simulink model "Distribution_v1"  (Simulink 7.9)
settings: Solver=VariableStepDiscrete  StartTime=0.0  StopTime=500  RelTol=1e-3
libraries: simeventslib x13
(part 1 of 2)
settings Model: Creator=tsprock3  LastModifiedBy=tsprock3
settings DebuggingCC: SimStateOlderReleaseMsg=warning

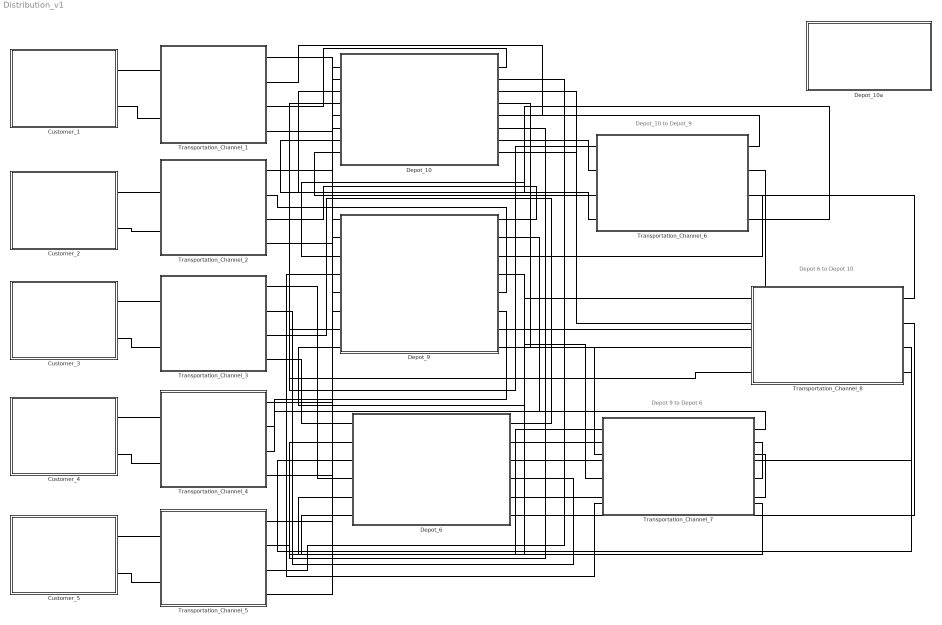
== system Distribution_v1 ==
  note: Depot_10 to Depot_9
  note: Depot 9 to Depot 6
  note: Depot 6 to Depot 10
  Customer_1 : Subsystem
  Customer_2 : Subsystem
  Customer_3 : Subsystem
  Customer_4 : Subsystem
  Customer_5 : Subsystem
  Depot_10 : Subsystem
  Depot_10a : Subsystem
  Depot_6 : Subsystem
  Depot_9 : Subsystem
  Transportation_Channel_1 : Subsystem
  Transportation_Channel_2 : Subsystem
  Transportation_Channel_3 : Subsystem
  Transportation_Channel_4 : Subsystem
  Transportation_Channel_5 : Subsystem
  Transportation_Channel_6 : Subsystem
  Transportation_Channel_7 : Subsystem
  Transportation_Channel_8 : Subsystem
  connections:
  Transportation_Channel_1/RConn4 -- Depot_10/LConn1
  Transportation_Channel_1/RConn3 -- Depot_10/RConn1
  Transportation_Channel_1/RConn1 -- Depot_10/LConn5
  Depot_10/RConn5 -- Transportation_Channel_1/RConn2
  Transportation_Channel_2/LConn2 -- Customer_2/RConn2
  Customer_2/RConn1 -- Transportation_Channel_2/LConn1
  Transportation_Channel_2/RConn1 -- Depot_9/LConn5
  Depot_9/RConn5 -- Transportation_Channel_2/RConn2
  Customer_3/RConn1 -- Transportation_Channel_3/LConn1
  Transportation_Channel_3/LConn2 -- Customer_3/RConn2
  Transportation_Channel_3/RConn1 -- Depot_6/LConn4
  Transportation_Channel_3/RConn2 -- Depot_6/RConn4
  Transportation_Channel_3/RConn3 -- Depot_6/RConn1
  Transportation_Channel_3/RConn4 -- Depot_6/LConn1
  Transportation_Channel_2/RConn3 -- Depot_9/RConn1
  Transportation_Channel_2/RConn4 -- Depot_9/LConn1
  Transportation_Channel_4/LConn2 -- Customer_4/RConn2
  Customer_4/RConn1 -- Transportation_Channel_4/LConn1
  Transportation_Channel_4/RConn1 -- Depot_9/LConn6
  Transportation_Channel_4/RConn3 -- Depot_9/RConn2
  Transportation_Channel_4/RConn4 -- Depot_9/LConn2
  Depot_9/RConn6 -- Transportation_Channel_4/RConn2
  Transportation_Channel_5/LConn2 -- Customer_5/RConn2
  Customer_5/RConn1 -- Transportation_Channel_5/LConn1
  Transportation_Channel_5/RConn1 -- Depot_10/LConn6
  Depot_10/RConn6 -- Transportation_Channel_5/RConn2
  Transportation_Channel_5/RConn3 -- Depot_10/RConn2
  Transportation_Channel_5/RConn4 -- Depot_10/LConn2
  Transportation_Channel_6/RConn3 -- Depot_9/RConn3
  Transportation_Channel_6/RConn4 -- Depot_9/LConn3
  Depot_10/RConn3 -- Transportation_Channel_6/LConn3
  Transportation_Channel_6/LConn4 -- Depot_10/LConn3
  Depot_6/RConn2 -- Transportation_Channel_7/RConn3
  Transportation_Channel_7/RConn4 -- Depot_6/LConn2
  Depot_9/RConn4 -- Transportation_Channel_7/LConn3
  Transportation_Channel_7/LConn4 -- Depot_9/LConn4
  Depot_6/RConn3 -- Transportation_Channel_8/RConn3
  Transportation_Channel_8/RConn4 -- Depot_6/LConn3
  Depot_10/LConn4 -- Transportation_Channel_8/LConn4
  Transportation_Channel_8/LConn3 -- Depot_10/RConn4
  Depot_10/RConn8 -- Transportation_Channel_8/LConn2
  Transportation_Channel_8/LConn1 -- Depot_6/LConn6
  Depot_6/RConn6 -- Transportation_Channel_8/RConn2
  Transportation_Channel_8/RConn1 -- Depot_10/LConn8
  Depot_10/RConn7 -- Transportation_Channel_6/LConn2
  Transportation_Channel_6/LConn1 -- Depot_9/LConn7
  Depot_9/RConn7 -- Transportation_Channel_6/RConn2
  Transportation_Channel_6/RConn1 -- Depot_10/LConn7
  Depot_9/RConn8 -- Transportation_Channel_7/LConn2
  Transportation_Channel_7/LConn1 -- Depot_6/LConn5
  Depot_6/RConn5 -- Transportation_Channel_7/RConn2
  Transportation_Channel_7/RConn1 -- Depot_9/LConn8
  Customer_1/RConn1 -- Transportation_Channel_1/LConn1
  Customer_1/RConn2 -- Transportation_Channel_1/LConn2

== system Distribution_v1/Customer_1 ==
  Clock : Clock
  Discrete Event Signal to Workspace : simeventslib/SimEvents Sinks/Discrete Event Signal to Workspace  VariableName=Customer_1  SaveFormat=Structure With Time  isMonitorOnly=off  isRecordIC=off
  Entity Sink : EntitySink
  Get Attribute : GetAttribute  AttributeName=Origin|Destination|Start  AttributeMissing=Error|Error|Error  AttributeDefaultValue=1|1|1  AttributeTreatAsVector=1|1|1  AttributeSendTiming=After entity departure|After entity departure|After entity departure  EvaluatedDefaultAttributeValue={[];[];[]}
      settings: OutputPortMap=o1,o2,o3
  Mux : Mux  Inputs=3
  Path Combiner : PathCombiner  NumberInputPorts=4
  Set Attribute : SetAttribute  AttributeName=Route|Origin|Destination|Start  AttributeFrom=Dialog|Dialog|Dialog|Signal port  AttributeValue=[1 10 9 2]|1|2|1  AttributeTreatAsVector=0|1|1|1  EvaluatedAttributeValue={[1 10 9 2];1;2;[]}
      settings: InputPortMap=u3
  Set Attribute1 : SetAttribute  AttributeName=Route|Origin|Destination|Start  AttributeFrom=Dialog|Dialog|Dialog|Signal port  AttributeValue=[1 10 6 3]|1|3|1  AttributeTreatAsVector=0|1|1|1  EvaluatedAttributeValue={[1 10 6 3];1;3;[]}
      settings: InputPortMap=u3
  Set Attribute2 : SetAttribute  AttributeName=Route|Origin|Destination|Start  AttributeFrom=Dialog|Dialog|Dialog|Signal port  AttributeValue=[1 10 5 0]|1|5|1  AttributeTreatAsVector=0|1|1|1  EvaluatedAttributeValue={[1 10 5 0];1;5;[]}
      settings: InputPortMap=u3
  Set Attribute3 : SetAttribute  AttributeName=Route|Origin|Destination|Start  AttributeFrom=Dialog|Dialog|Dialog|Signal port  AttributeValue=[1 10 9 4]|1|4|1  AttributeTreatAsVector=0|1|1|1  EvaluatedAttributeValue={[1 10 9 4];1;4;[]}
      settings: InputPortMap=u3
  Timed to Event Signal : TimedToEventSignal
  To_Customer_2 : TimeBasedEntityGenerator  Distribution=Exponential  InitialSeed=18340  Mean=1000/913  GenerateEntityAtSimulationStart=off
  To_Customer_3 : TimeBasedEntityGenerator  Distribution=Exponential  InitialSeed=13103  Mean=1000/105  GenerateEntityAtSimulationStart=off
  To_Customer_4 : TimeBasedEntityGenerator  Distribution=Exponential  InitialSeed=21557  Mean=1000/746  GenerateEntityAtSimulationStart=off
  To_Customer_5 : TimeBasedEntityGenerator  Distribution=Exponential  InitialSeed=24774  Mean=1000/737  GenerateEntityAtSimulationStart=off
  OUT_Shipment_1 : PMIOPort  Port=1  Side=Right
  IN_Shipment_1 : PMIOPort  Port=2  Side=Right
  wires:
  Clock/1 -> Timed to Event Signal/1
  Timed to Event Signal/1 -> Set Attribute/1, Set Attribute1/1, Set Attribute3/1, Set Attribute2/1
  Get Attribute/1 -> Mux/1
  Get Attribute/2 -> Mux/2
  Get Attribute/3 -> Mux/3
  Mux/1 -> Discrete Event Signal to Workspace/1
  connections:
  OUT_Shipment_1/RConn1 -- Path Combiner/RConn1
  To_Customer_2/RConn1 -- Set Attribute/LConn1
  To_Customer_3/RConn1 -- Set Attribute1/LConn1
  To_Customer_5/RConn1 -- Set Attribute2/LConn1
  To_Customer_4/RConn1 -- Set Attribute3/LConn1
  Set Attribute/RConn1 -- Path Combiner/LConn1
  Set Attribute1/RConn1 -- Path Combiner/LConn2
  Set Attribute3/RConn1 -- Path Combiner/LConn3
  Set Attribute2/RConn1 -- Path Combiner/LConn4
  Get Attribute/LConn1 -- IN_Shipment_1/RConn1
  Entity Sink/LConn1 -- Get Attribute/RConn1

== system Distribution_v1/Customer_2 ==
  Clock : Clock
  Discrete Event Signal to Workspace : simeventslib/SimEvents Sinks/Discrete Event Signal to Workspace  VariableName=Customer_2  SaveFormat=Structure With Time  isMonitorOnly=off  isRecordIC=off
  Entity Sink : EntitySink
  Get Attribute : GetAttribute  AttributeName=Origin|Destination|Start  AttributeMissing=Error|Error|Error  AttributeDefaultValue=1|1|1  AttributeTreatAsVector=1|1|1  AttributeSendTiming=After entity departure|After entity departure|After entity departure  EvaluatedDefaultAttributeValue={[];[];[]}
      settings: OutputPortMap=o1,o2,o3
  Mux : Mux  Inputs=3
  Path Combiner : PathCombiner  NumberInputPorts=4
  Set Attribute : SetAttribute  AttributeName=Route|Origin|Destination|Start  AttributeFrom=Dialog|Dialog|Dialog|Signal port  AttributeValue=[2 9 10 1]|2|1|1  AttributeTreatAsVector=0|1|1|1  EvaluatedAttributeValue={[2 9 10 1];2;1;[]}
      settings: InputPortMap=u3
  Set Attribute1 : SetAttribute  AttributeName=Route|Origin|Destination|Start  AttributeFrom=Dialog|Dialog|Dialog|Signal port  AttributeValue=[2 9 6 3]|2|3|1  AttributeTreatAsVector=0|1|1|1  EvaluatedAttributeValue={[2 9 6 3];2;3;[]}
      settings: InputPortMap=u3
  Set Attribute2 : SetAttribute  AttributeName=Route|Origin|Destination|Start  AttributeFrom=Dialog|Dialog|Dialog|Signal port  AttributeValue=[2 9 10 5]|2|5|1  AttributeTreatAsVector=0|1|1|1  EvaluatedAttributeValue={[2 9 10 5];2;5;[]}
      settings: InputPortMap=u3
  Set Attribute3 : SetAttribute  AttributeName=Route|Origin|Destination|Start  AttributeFrom=Dialog|Dialog|Dialog|Signal port  AttributeValue=[2 9 4 0]|2|4|1  AttributeTreatAsVector=0|1|1|1  EvaluatedAttributeValue={[2 9 4 0];2;4;[]}
      settings: InputPortMap=u3
  Timed to Event Signal : TimedToEventSignal
  To_Customer_1 : TimeBasedEntityGenerator  Distribution=Exponential  InitialSeed=27991  Mean=1000/562  GenerateEntityAtSimulationStart=off
  To_Customer_3 : TimeBasedEntityGenerator  Distribution=Exponential  InitialSeed=16319  Mean=1000/185  GenerateEntityAtSimulationStart=off
  To_Customer_4 : TimeBasedEntityGenerator  Distribution=Exponential  InitialSeed=31208  Mean=1000/598  GenerateEntityAtSimulationStart=off
  To_Customer_5 : TimeBasedEntityGenerator  Distribution=Exponential  InitialSeed=34425  Mean=1000/300  GenerateEntityAtSimulationStart=off
  OUT_Shipment_1 : PMIOPort  Port=1  Side=Right
  IN_Shipment_1 : PMIOPort  Port=2  Side=Right
  wires:
  Clock/1 -> Timed to Event Signal/1
  Get Attribute/1 -> Mux/1
  Get Attribute/2 -> Mux/2
  Get Attribute/3 -> Mux/3
  Mux/1 -> Discrete Event Signal to Workspace/1
  Timed to Event Signal/1 -> Set Attribute/1, Set Attribute1/1, Set Attribute3/1, Set Attribute2/1
  connections:
  OUT_Shipment_1/RConn1 -- Path Combiner/RConn1
  To_Customer_1/RConn1 -- Set Attribute/LConn1
  To_Customer_3/RConn1 -- Set Attribute1/LConn1
  To_Customer_5/RConn1 -- Set Attribute2/LConn1
  To_Customer_4/RConn1 -- Set Attribute3/LConn1
  Set Attribute/RConn1 -- Path Combiner/LConn1
  Set Attribute1/RConn1 -- Path Combiner/LConn2
  Set Attribute3/RConn1 -- Path Combiner/LConn3
  Set Attribute2/RConn1 -- Path Combiner/LConn4
  Entity Sink/LConn1 -- Get Attribute/RConn1
  Get Attribute/LConn1 -- IN_Shipment_1/RConn1

== system Distribution_v1/Customer_3 ==
  Clock : Clock
  Discrete Event Signal to Workspace : simeventslib/SimEvents Sinks/Discrete Event Signal to Workspace  VariableName=Customer_3  SaveFormat=Structure With Time  isMonitorOnly=off  isRecordIC=off
  Entity Sink : EntitySink
  Get Attribute : GetAttribute  AttributeName=Origin|Destination|Start  AttributeMissing=Error|Error|Error  AttributeDefaultValue=1|1|1  AttributeTreatAsVector=1|1|1  AttributeSendTiming=After entity departure|After entity departure|After entity departure  EvaluatedDefaultAttributeValue={[];[];[]}
      settings: OutputPortMap=o1,o2,o3
  Mux : Mux  Inputs=3
  Path Combiner : PathCombiner  NumberInputPorts=4
  Set Attribute : SetAttribute  AttributeName=Route|Origin|Destination|Start  AttributeFrom=Dialog|Dialog|Dialog|Signal port  AttributeValue=[3 6 10 1]|3|1|1  AttributeTreatAsVector=0|1|1|1  EvaluatedAttributeValue={[3 6 10 1];3;1;[]}
      settings: InputPortMap=u3
  Set Attribute1 : SetAttribute  AttributeName=Route|Origin|Destination|Start  AttributeFrom=Dialog|Dialog|Dialog|Signal port  AttributeValue=[3 6 9 2]|3|2|1  AttributeTreatAsVector=0|1|1|1  EvaluatedAttributeValue={[3 6 9 2];3;2;[]}
      settings: InputPortMap=u3
  Set Attribute2 : SetAttribute  AttributeName=Route|Origin|Destination|Start  AttributeFrom=Dialog|Dialog|Dialog|Signal port  AttributeValue=[3 6 10 5]|3|5|1  AttributeTreatAsVector=0|1|1|1  EvaluatedAttributeValue={[3 6 10 5];3;5;[]}
      settings: InputPortMap=u3
  Set Attribute3 : SetAttribute  AttributeName=Route|Origin|Destination|Start  AttributeFrom=Dialog|Dialog|Dialog|Signal port  AttributeValue=[3 6 9 4]|3|4|1  AttributeTreatAsVector=0|1|1|1  EvaluatedAttributeValue={[3 6 9 4];3;4;[]}
      settings: InputPortMap=u3
  Timed to Event Signal : TimedToEventSignal
  To_Customer_1 : TimeBasedEntityGenerator  Distribution=Exponential  InitialSeed=37642  Mean=1000/135  GenerateEntityAtSimulationStart=off
  To_Customer_2 : TimeBasedEntityGenerator  Distribution=Exponential  InitialSeed=19536  Mean=1000/213  GenerateEntityAtSimulationStart=off
  To_Customer_4 : TimeBasedEntityGenerator  Distribution=Exponential  InitialSeed=40859  Mean=1000/895  GenerateEntityAtSimulationStart=off
  To_Customer_5 : TimeBasedEntityGenerator  Distribution=Exponential  InitialSeed=44076  Mean=1000/72  GenerateEntityAtSimulationStart=off
  OUT_Shipment_1 : PMIOPort  Port=1  Side=Right
  IN_Shipment_1 : PMIOPort  Port=2  Side=Right
  wires:
  Clock/1 -> Timed to Event Signal/1
  Get Attribute/1 -> Mux/1
  Get Attribute/2 -> Mux/2
  Get Attribute/3 -> Mux/3
  Mux/1 -> Discrete Event Signal to Workspace/1
  Timed to Event Signal/1 -> Set Attribute/1, Set Attribute1/1, Set Attribute3/1, Set Attribute2/1
  connections:
  OUT_Shipment_1/RConn1 -- Path Combiner/RConn1
  To_Customer_1/RConn1 -- Set Attribute/LConn1
  To_Customer_2/RConn1 -- Set Attribute1/LConn1
  To_Customer_5/RConn1 -- Set Attribute2/LConn1
  To_Customer_4/RConn1 -- Set Attribute3/LConn1
  Set Attribute/RConn1 -- Path Combiner/LConn1
  Set Attribute1/RConn1 -- Path Combiner/LConn2
  Set Attribute3/RConn1 -- Path Combiner/LConn3
  Set Attribute2/RConn1 -- Path Combiner/LConn4
  Get Attribute/LConn1 -- IN_Shipment_1/RConn1
  Entity Sink/LConn1 -- Get Attribute/RConn1

== system Distribution_v1/Customer_4 ==
  Clock : Clock
  Discrete Event Signal to Workspace : simeventslib/SimEvents Sinks/Discrete Event Signal to Workspace  VariableName=Customer_4  SaveFormat=Structure With Time  isMonitorOnly=off  isRecordIC=off
  Entity Sink : EntitySink
  Get Attribute : GetAttribute  AttributeName=Origin|Destination|Start  AttributeMissing=Error|Error|Error  AttributeDefaultValue=1|1|1  AttributeTreatAsVector=1|1|1  AttributeSendTiming=After entity departure|After entity departure|After entity departure  EvaluatedDefaultAttributeValue={[];[];[]}
      settings: OutputPortMap=o1,o2,o3
  Mux : Mux  Inputs=3
  Path Combiner : PathCombiner  NumberInputPorts=4
  Set Attribute : SetAttribute  AttributeName=Route|Origin|Destination|Start  AttributeFrom=Dialog|Dialog|Dialog|Signal port  AttributeValue=[4 9 10 1]|4|1|1  AttributeTreatAsVector=0|1|1|1  EvaluatedAttributeValue={[4 9 10 1];4;1;[]}
      settings: InputPortMap=u3
  Set Attribute1 : SetAttribute  AttributeName=Route|Origin|Destination|Start  AttributeFrom=Dialog|Dialog|Dialog|Signal port  AttributeValue=[4 9 2 0]|4|2|1  AttributeTreatAsVector=0|1|1|1  EvaluatedAttributeValue={[4 9 2 0];4;2;[]}
      settings: InputPortMap=u3
  Set Attribute2 : SetAttribute  AttributeName=Route|Origin|Destination|Start  AttributeFrom=Dialog|Dialog|Dialog|Signal port  AttributeValue=[4 9 10 5]|4|5|1  AttributeTreatAsVector=0|1|1|1  EvaluatedAttributeValue={[4 9 10 5];4;5;[]}
      settings: InputPortMap=u3
  Set Attribute3 : SetAttribute  AttributeName=Route|Origin|Destination|Start  AttributeFrom=Dialog|Dialog|Dialog|Signal port  AttributeValue=[4 9 6 3]|4|3|1  AttributeTreatAsVector=0|1|1|1  EvaluatedAttributeValue={[4 9 6 3];4;3;[]}
      settings: InputPortMap=u3
  Timed to Event Signal : TimedToEventSignal
  To_Customer_1 : TimeBasedEntityGenerator  Distribution=Exponential  InitialSeed=47293  Mean=1000/243  GenerateEntityAtSimulationStart=off
  To_Customer_2 : TimeBasedEntityGenerator  Distribution=Exponential  InitialSeed=22753  Mean=1000/54  GenerateEntityAtSimulationStart=off
  To_Customer_3 : TimeBasedEntityGenerator  Distribution=Exponential  InitialSeed=50510  Mean=1000/442  GenerateEntityAtSimulationStart=off
  To_Customer_5 : TimeBasedEntityGenerator  Distribution=Exponential  InitialSeed=53727  Mean=1000/14  GenerateEntityAtSimulationStart=off
  OUT_Shipment_1 : PMIOPort  Port=1  Side=Right
  IN_Shipment_1 : PMIOPort  Port=2  Side=Right
  wires:
  Clock/1 -> Timed to Event Signal/1
  Timed to Event Signal/1 -> Set Attribute3/1, Set Attribute/1, Set Attribute1/1, Set Attribute2/1
  Get Attribute/1 -> Mux/1
  Get Attribute/2 -> Mux/2
  Get Attribute/3 -> Mux/3
  Mux/1 -> Discrete Event Signal to Workspace/1
  connections:
  OUT_Shipment_1/RConn1 -- Path Combiner/RConn1
  To_Customer_1/RConn1 -- Set Attribute/LConn1
  To_Customer_2/RConn1 -- Set Attribute1/LConn1
  To_Customer_5/RConn1 -- Set Attribute2/LConn1
  To_Customer_3/RConn1 -- Set Attribute3/LConn1
  Set Attribute/RConn1 -- Path Combiner/LConn1
  Set Attribute1/RConn1 -- Path Combiner/LConn2
  Set Attribute3/RConn1 -- Path Combiner/LConn3
  Set Attribute2/RConn1 -- Path Combiner/LConn4
  Entity Sink/LConn1 -- Get Attribute/RConn1
  Get Attribute/LConn1 -- IN_Shipment_1/RConn1

== system Distribution_v1/Customer_5 ==
  Clock : Clock
  Discrete Event Signal to Workspace : simeventslib/SimEvents Sinks/Discrete Event Signal to Workspace  VariableName=Customer_5  SaveFormat=Structure With Time  isMonitorOnly=off  isRecordIC=off
  Entity Sink : EntitySink
  Get Attribute : GetAttribute  AttributeName=Origin|Destination|Start  AttributeMissing=Error|Error|Error  AttributeDefaultValue=1|1|1  AttributeTreatAsVector=1|1|1  AttributeSendTiming=After entity departure|After entity departure|After entity departure  EvaluatedDefaultAttributeValue={[];[];[]}
      settings: OutputPortMap=o1,o2,o3
  Mux : Mux  Inputs=3
  Path Combiner : PathCombiner  NumberInputPorts=4
  Set Attribute : SetAttribute  AttributeName=Route|Origin|Destination|Start  AttributeFrom=Dialog|Dialog|Dialog|Signal port  AttributeValue=[5 10 1 0]|5|1|1  AttributeTreatAsVector=0|1|1|1  EvaluatedAttributeValue={[5 10 1 0];5;1;[]}
      settings: InputPortMap=u3
  Set Attribute1 : SetAttribute  AttributeName=Route|Origin|Destination|Start  AttributeFrom=Dialog|Dialog|Dialog|Signal port  AttributeValue=[5 10 9 2]|5|2|1  AttributeTreatAsVector=0|1|1|1  EvaluatedAttributeValue={[5 10 9 2];5;2;[]}
      settings: InputPortMap=u3
  Set Attribute2 : SetAttribute  AttributeName=Route|Origin|Destination|Start  AttributeFrom=Dialog|Dialog|Dialog|Signal port  AttributeValue=[5 10 9 4]|5|4|1  AttributeTreatAsVector=0|1|1|1  EvaluatedAttributeValue={[5 10 9 4];5;4;[]}
      settings: InputPortMap=u3
  Set Attribute3 : SetAttribute  AttributeName=Route|Origin|Destination|Start  AttributeFrom=Dialog|Dialog|Dialog|Signal port  AttributeValue=[5 10 6 3]|5|3|1  AttributeTreatAsVector=0|1|1|1  EvaluatedAttributeValue={[5 10 6 3];5;3;[]}
      settings: InputPortMap=u3
  Timed to Event Signal : TimedToEventSignal
  To_Customer_1 : TimeBasedEntityGenerator  Distribution=Exponential  InitialSeed=56944  Mean=1000/898  GenerateEntityAtSimulationStart=off
  To_Customer_2 : TimeBasedEntityGenerator  Distribution=Exponential  InitialSeed=25970  Mean=1000/197  GenerateEntityAtSimulationStart=off
  To_Customer_3 : TimeBasedEntityGenerator  Distribution=Exponential  InitialSeed=60161  Mean=1000/94  GenerateEntityAtSimulationStart=off
  To_Customer_4 : TimeBasedEntityGenerator  Distribution=Exponential  InitialSeed=63378  Mean=1000/308  GenerateEntityAtSimulationStart=off
  OUT_Shipment_1 : PMIOPort  Port=1  Side=Right
  IN_Shipment_1 : PMIOPort  Port=2  Side=Right
  wires:
  Clock/1 -> Timed to Event Signal/1
  Timed to Event Signal/1 -> Set Attribute/1, Set Attribute1/1, Set Attribute3/1, Set Attribute2/1
  Get Attribute/1 -> Mux/1
  Get Attribute/2 -> Mux/2
  Get Attribute/3 -> Mux/3
  Mux/1 -> Discrete Event Signal to Workspace/1
  connections:
  OUT_Shipment_1/RConn1 -- Path Combiner/RConn1
  To_Customer_1/RConn1 -- Set Attribute/LConn1
  To_Customer_2/RConn1 -- Set Attribute1/LConn1
  To_Customer_4/RConn1 -- Set Attribute2/LConn1
  To_Customer_3/RConn1 -- Set Attribute3/LConn1
  Set Attribute/RConn1 -- Path Combiner/LConn1
  Set Attribute1/RConn1 -- Path Combiner/LConn2
  Set Attribute3/RConn1 -- Path Combiner/LConn3
  Set Attribute2/RConn1 -- Path Combiner/LConn4
  Get Attribute/LConn1 -- IN_Shipment_1/RConn1
  Entity Sink/LConn1 -- Get Attribute/RConn1

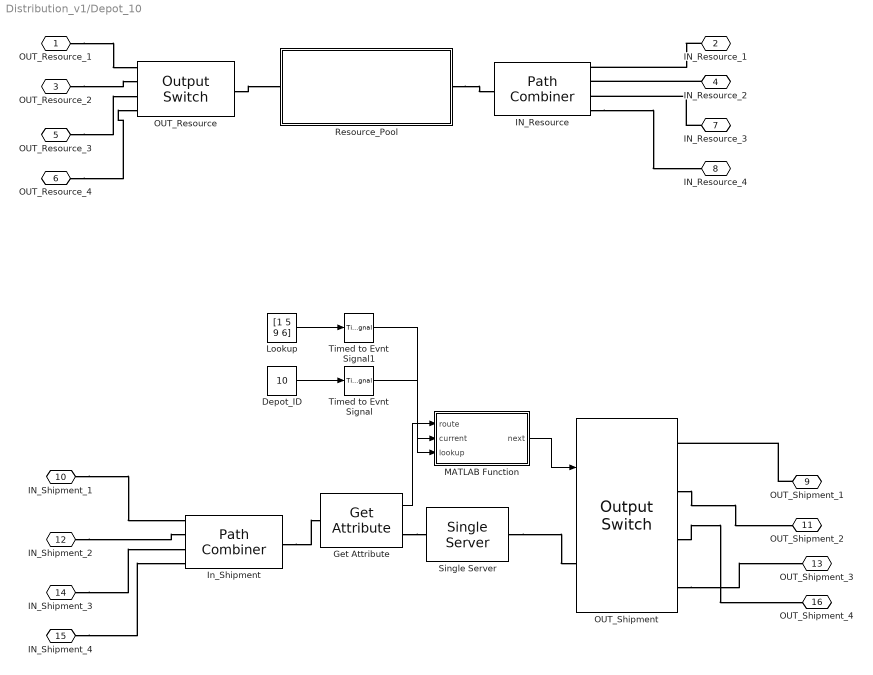
== system Distribution_v1/Depot_10 ==
  Depot_ID : Constant  Value=10
  Get Attribute : GetAttribute  AttributeName=Route  EvaluatedDefaultAttributeValue={[]}
      settings: OutputPortMap=o1
  IN_Resource : PathCombiner  NumberInputPorts=4
  In_Shipment : PathCombiner  NumberInputPorts=4
  Lookup : Constant  Value=[1 5 9 6]
  MATLAB Function : MATLAB Function  TreatAsAtomicUnit=on
  OUT_Resource : OutputSwitch  NumberOutputPorts=4  SwitchingCriterion=Round robin  InitialSeed=57769
  OUT_Shipment : OutputSwitch  NumberOutputPorts=4  SwitchingCriterion=From signal port p  AttributeName=Customer
  Resource_Pool : Subsystem  mask{Quantity=6}
      mask prompts: Quantity "How many entities in resource pool?"
  Single Server : SingleServer  ServiceTime=0
  Timed to Evnt Signal : TimedToEventSignal
  Timed to Evnt Signal1 : TimedToEventSignal
  OUT_Resource_1 : PMIOPort  Port=1  Side=Right
  IN_Resource_1 : PMIOPort  Port=2  Side=Left
  OUT_Resource_2 : PMIOPort  Port=3  Side=Right
  IN_Resource_2 : PMIOPort  Port=4  Side=Left
  OUT_Resource_3 : PMIOPort  Port=5  Side=Right
  OUT_Resource_4 : PMIOPort  Port=6  Side=Right
  IN_Resource_3 : PMIOPort  Port=7  Side=Left
  IN_Resource_4 : PMIOPort  Port=8  Side=Left
  OUT_Shipment_1 : PMIOPort  Port=9  Side=Right
  IN_Shipment_1 : PMIOPort  Port=10  Side=Left
  OUT_Shipment_2 : PMIOPort  Port=11  Side=Right
  IN_Shipment_2 : PMIOPort  Port=12  Side=Left
  OUT_Shipment_3 : PMIOPort  Port=13  Side=Right
  IN_Shipment_3 : PMIOPort  Port=14  Side=Left
  IN_Shipment_4 : PMIOPort  Port=15  Side=Left
  OUT_Shipment_4 : PMIOPort  Port=16  Side=Right
  wires:
  Depot_ID/1 -> Timed to Evnt Signal/1
  MATLAB Function/1(next) -> OUT_Shipment/1
  Get Attribute/1 -> MATLAB Function/1(route)
  Timed to Evnt Signal/1 -> MATLAB Function/2(current)
  Lookup/1 -> Timed to Evnt Signal1/1
  Timed to Evnt Signal1/1 -> MATLAB Function/3(lookup)
  connections:
  OUT_Resource/LConn1 -- Resource_Pool/LConn1
  Resource_Pool/RConn1 -- IN_Resource/RConn1
  OUT_Resource_1/RConn1 -- OUT_Resource/RConn1
  IN_Resource_1/RConn1 -- IN_Resource/LConn1
  OUT_Resource_2/RConn1 -- OUT_Resource/RConn2
  IN_Resource_2/RConn1 -- IN_Resource/LConn2
  OUT_Resource_3/RConn1 -- OUT_Resource/RConn3
  IN_Resource_3/RConn1 -- IN_Resource/LConn3
  OUT_Shipment_1/RConn1 -- OUT_Shipment/RConn1
  IN_Shipment_1/RConn1 -- In_Shipment/LConn1
  IN_Shipment_2/RConn1 -- In_Shipment/LConn2
  IN_Shipment_3/RConn1 -- In_Shipment/LConn3
  In_Shipment/RConn1 -- Get Attribute/LConn1
  Get Attribute/RConn1 -- Single Server/LConn1
  Single Server/RConn1 -- OUT_Shipment/LConn1
  OUT_Shipment/RConn2 -- OUT_Shipment_2/RConn1
  OUT_Resource_4/RConn1 -- OUT_Resource/RConn4
  IN_Resource/LConn4 -- IN_Resource_4/RConn1
  IN_Shipment_4/RConn1 -- In_Shipment/LConn4
  OUT_Shipment/RConn3 -- OUT_Shipment_4/RConn1
  OUT_Shipment/RConn4 -- OUT_Shipment_3/RConn1

== system Distribution_v1/Depot_10a ==
  Control: Resource Allocation : MATLAB Function  TreatAsAtomicUnit=on
  Get Attribute : GetAttribute  AttributeName=Route  EvaluatedDefaultAttributeValue={[]}
      settings: OutputPortMap=o1
  IN_Resource : PathCombiner  NumberInputPorts=4
  In_Shipment : PathCombiner  NumberInputPorts=4
  Lookup : Constant  Value=[1 5 9 6]
  MATLAB Function : MATLAB Function  TreatAsAtomicUnit=on
  Node_ID : Constant  Value=10
  OUT_Resource : OutputSwitch  NumberOutputPorts=2  SwitchingCriterion=From signal port p  InitialSeed=57769
  OUT_Shipment : OutputSwitch  NumberOutputPorts=2  SwitchingCriterion=From signal port p  AttributeName=Customer
  Resource_Pool : Subsystem  mask{Quantity=6}
      mask prompts: Quantity "How many entities in resource pool?"
  Single Server : SingleServer  ServiceTime=0
  Timed to Evnt Signal : TimedToEventSignal
  Timed to Evnt Signal1 : TimedToEventSignal
  OUT_Resource_1 : PMIOPort  Port=1  Side=Right
  OUT_Shipment_1 : PMIOPort  Port=2  Side=Right
  OUT_Shipment_2 : PMIOPort  Port=3  Side=Right
  OUT_Resource_2 : PMIOPort  Port=4  Side=Right
  wires:
  Control: Resource Allocation/1(OUT_1) -> OUT_Resource/1
  [TC6_Metrics] -> Control: Resource Allocation/4(IN_4)
  [TC8_Metrics] -> Control: Resource Allocation/3(IN_3)
  [TC5_Metrics] -> Control: Resource Allocation/2(IN_2)
  [TC1_Metrics] -> Control: Resource Allocation/1(IN_1)
  Timed to Evnt Signal1/1 -> MATLAB Function/3(lookup)
  Lookup/1 -> Timed to Evnt Signal1/1
  Timed to Evnt Signal/1 -> MATLAB Function/2(current)
  Get Attribute/1 -> MATLAB Function/1(route)
  MATLAB Function/1(next) -> OUT_Shipment/1
  Node_ID/1 -> Timed to Evnt Signal/1
  connections:
  Single Server/RConn1 -- OUT_Shipment/LConn1
  Get Attribute/RConn1 -- Single Server/LConn1
  In_Shipment/RConn1 -- Get Attribute/LConn1
  Resource_Pool/RConn1 -- IN_Resource/RConn1
  OUT_Resource/LConn1 -- Resource_Pool/LConn1
  OUT_Resource/RConn1 -- OUT_Resource_1/RConn1
  OUT_Shipment/RConn1 -- OUT_Shipment_1/RConn1
  OUT_Shipment/RConn2 -- OUT_Shipment_2/RConn1
  OUT_Resource/RConn2 -- OUT_Resource_2/RConn1

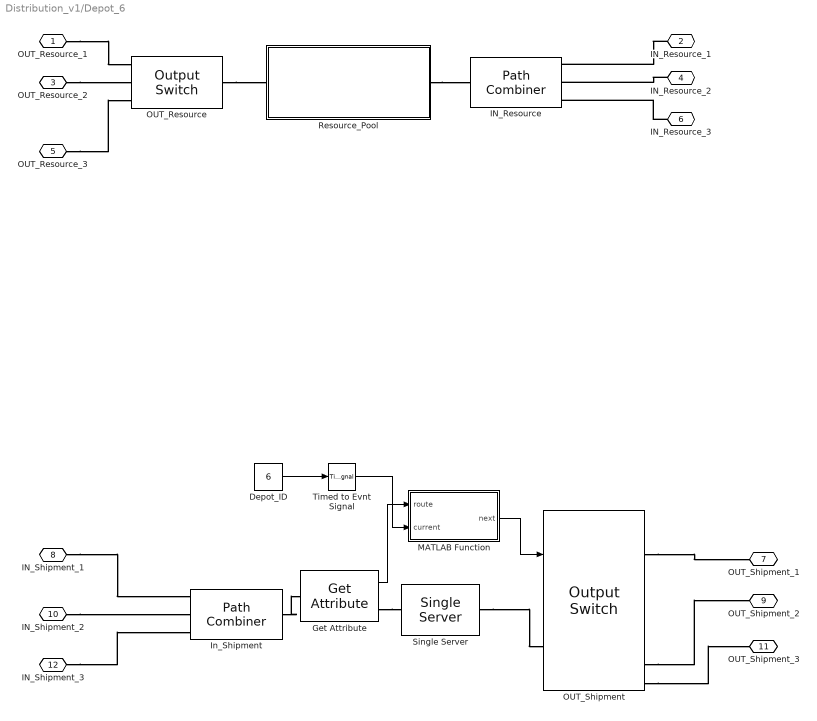
== system Distribution_v1/Depot_6 ==
  Depot_ID : Constant  Value=6
  Get Attribute : GetAttribute  AttributeName=Route  EvaluatedDefaultAttributeValue={[]}
      settings: OutputPortMap=o1
  IN_Resource : PathCombiner
  In_Shipment : PathCombiner
  MATLAB Function : MATLAB Function  TreatAsAtomicUnit=on
  OUT_Resource : OutputSwitch  SwitchingCriterion=Round robin  InitialSeed=60986
  OUT_Shipment : OutputSwitch  NumberOutputPorts=10  SwitchingCriterion=From signal port p  AttributeName=Customer
  Resource_Pool : Subsystem  mask{Quantity=2}
      mask prompts: Quantity "How many entities in resource pool?"
  Single Server : SingleServer  ServiceTime=0
  Timed to Evnt Signal : TimedToEventSignal
  OUT_Resource_1 : PMIOPort  Port=1  Side=Right
  IN_Resource_1 : PMIOPort  Port=2  Side=Left
  OUT_Resource_2 : PMIOPort  Port=3  Side=Right
  IN_Resource_2 : PMIOPort  Port=4  Side=Left
  OUT_Resource_3 : PMIOPort  Port=5  Side=Right
  IN_Resource_3 : PMIOPort  Port=6  Side=Left
  OUT_Shipment_1 : PMIOPort  Port=7  Side=Right
  IN_Shipment_1 : PMIOPort  Port=8  Side=Left
  OUT_Shipment_2 : PMIOPort  Port=9  Side=Right
  IN_Shipment_2 : PMIOPort  Port=10  Side=Left
  OUT_Shipment_3 : PMIOPort  Port=11  Side=Right
  IN_Shipment_3 : PMIOPort  Port=12  Side=Left
  wires:
  Depot_ID/1 -> Timed to Evnt Signal/1
  MATLAB Function/1(next) -> OUT_Shipment/1
  Get Attribute/1 -> MATLAB Function/1(route)
  Timed to Evnt Signal/1 -> MATLAB Function/2(current)
  connections:
  OUT_Resource/LConn1 -- Resource_Pool/LConn1
  Resource_Pool/RConn1 -- IN_Resource/RConn1
  OUT_Resource_1/RConn1 -- OUT_Resource/RConn1
  IN_Resource_1/RConn1 -- IN_Resource/LConn1
  OUT_Resource_2/RConn1 -- OUT_Resource/RConn2
  IN_Resource_2/RConn1 -- IN_Resource/LConn2
  OUT_Resource_3/RConn1 -- OUT_Resource/RConn3
  IN_Resource_3/RConn1 -- IN_Resource/LConn3
  IN_Shipment_1/RConn1 -- In_Shipment/LConn1
  IN_Shipment_2/RConn1 -- In_Shipment/LConn2
  IN_Shipment_3/RConn1 -- In_Shipment/LConn3
  In_Shipment/RConn1 -- Get Attribute/LConn1
  Get Attribute/RConn1 -- Single Server/LConn1
  Single Server/RConn1 -- OUT_Shipment/LConn1
  OUT_Shipment/RConn3 -- OUT_Shipment_1/RConn1
  OUT_Shipment/RConn9 -- OUT_Shipment_2/RConn1
  OUT_Shipment/RConn10 -- OUT_Shipment_3/RConn1

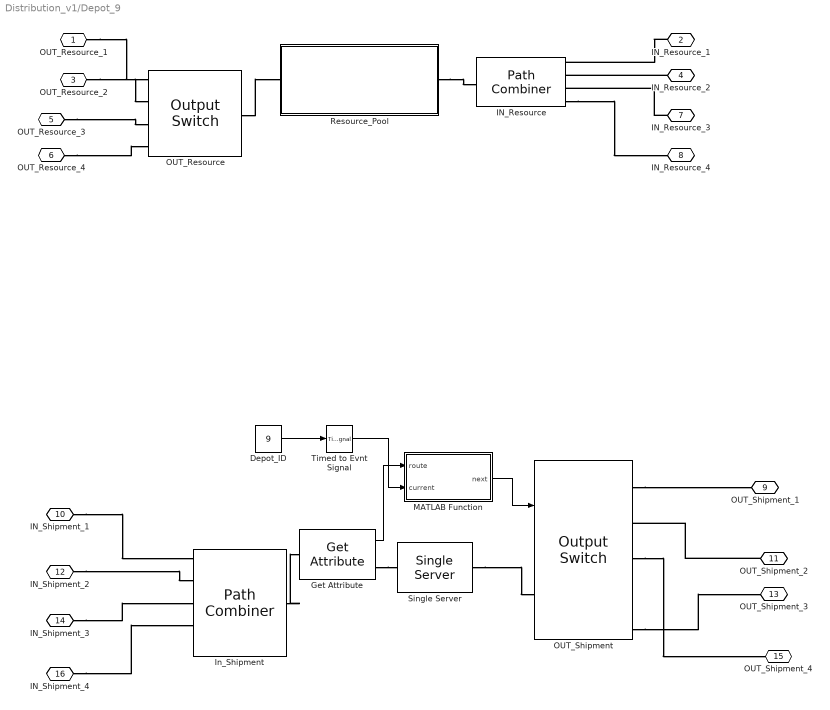
== system Distribution_v1/Depot_9 ==
  Depot_ID : Constant  Value=9
  Get Attribute : GetAttribute  AttributeName=Route  EvaluatedDefaultAttributeValue={[]}
      settings: OutputPortMap=o1
  IN_Resource : PathCombiner  NumberInputPorts=4
  In_Shipment : PathCombiner  NumberInputPorts=5
  MATLAB Function : MATLAB Function  TreatAsAtomicUnit=on
  OUT_Resource : OutputSwitch  NumberOutputPorts=4  SwitchingCriterion=Round robin  InitialSeed=64203
  OUT_Shipment : OutputSwitch  NumberOutputPorts=10  SwitchingCriterion=From signal port p  AttributeName=Customer
  Resource_Pool : Subsystem  mask{Quantity=6}
      mask prompts: Quantity "How many entities in resource pool?"
  Single Server : SingleServer  ServiceTime=0
  Timed to Evnt Signal : TimedToEventSignal
  OUT_Resource_1 : PMIOPort  Port=1  Side=Right
  IN_Resource_1 : PMIOPort  Port=2  Side=Left
  OUT_Resource_2 : PMIOPort  Port=3  Side=Right
  IN_Resource_2 : PMIOPort  Port=4  Side=Left
  OUT_Resource_3 : PMIOPort  Port=5  Side=Right
  OUT_Resource_4 : PMIOPort  Port=6  Side=Right
  IN_Resource_3 : PMIOPort  Port=7  Side=Left
  IN_Resource_4 : PMIOPort  Port=8  Side=Left
  OUT_Shipment_1 : PMIOPort  Port=9  Side=Right
  IN_Shipment_1 : PMIOPort  Port=10  Side=Left
  OUT_Shipment_2 : PMIOPort  Port=11  Side=Right
  IN_Shipment_2 : PMIOPort  Port=12  Side=Left
  OUT_Shipment_3 : PMIOPort  Port=13  Side=Right
  IN_Shipment_3 : PMIOPort  Port=14  Side=Left
  OUT_Shipment_4 : PMIOPort  Port=15  Side=Right
  IN_Shipment_4 : PMIOPort  Port=16  Side=Left
  wires:
  Depot_ID/1 -> Timed to Evnt Signal/1
  MATLAB Function/1(next) -> OUT_Shipment/1
  Get Attribute/1 -> MATLAB Function/1(route)
  Timed to Evnt Signal/1 -> MATLAB Function/2(current)
  connections:
  OUT_Resource/LConn1 -- Resource_Pool/LConn1
  Resource_Pool/RConn1 -- IN_Resource/RConn1
  OUT_Resource_1/RConn1 -- OUT_Resource/RConn1
  IN_Resource_1/RConn1 -- IN_Resource/LConn1
  OUT_Resource_2/RConn1 -- OUT_Resource/RConn2
  IN_Resource_2/RConn1 -- IN_Resource/LConn2
  OUT_Resource_3/RConn1 -- OUT_Resource/RConn3
  IN_Resource_3/RConn1 -- IN_Resource/LConn3
  IN_Shipment_1/RConn1 -- In_Shipment/LConn1
  IN_Shipment_2/RConn1 -- In_Shipment/LConn2
  IN_Shipment_3/RConn1 -- In_Shipment/LConn3
  In_Shipment/RConn1 -- Get Attribute/LConn1
  Get Attribute/RConn1 -- Single Server/LConn1
  Single Server/RConn1 -- OUT_Shipment/LConn1
  OUT_Shipment/RConn2 -- OUT_Shipment_1/RConn1
  OUT_Shipment_2/RConn1 -- OUT_Shipment/RConn4
  OUT_Shipment/RConn10 -- OUT_Shipment_3/RConn1
  OUT_Shipment/RConn6 -- OUT_Shipment_4/RConn1
  IN_Shipment_4/RConn1 -- In_Shipment/LConn4
  OUT_Resource_4/RConn1 -- OUT_Resource/RConn4
  IN_Resource/LConn4 -- IN_Resource_4/RConn1

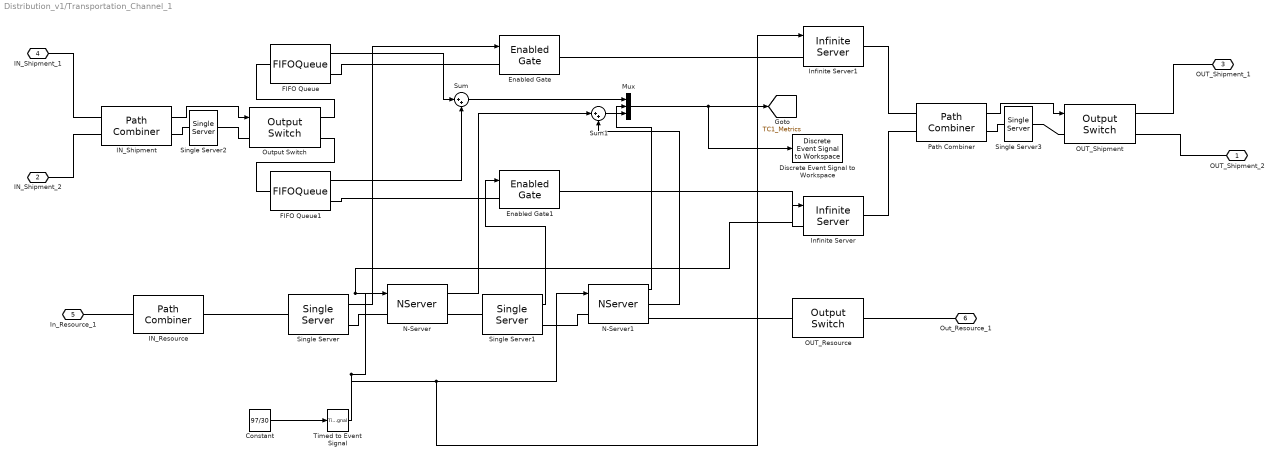
== system Distribution_v1/Transportation_Channel_1 ==
  Constant : Constant  Value=97/30
  Discrete Event Signal to Workspace : simeventslib/SimEvents Sinks/Discrete Event Signal to Workspace  VariableName=TC1_Status  SaveFormat=Structure With Time  isMonitorOnly=off  isRecordIC=off
  Enabled Gate : EnabledGate
  Enabled Gate1 : EnabledGate
  FIFO Queue : FIFOQueue  Capacity=inf  StatNumberInBlock=on
      settings: OutputPortMap=o1
  FIFO Queue1 : FIFOQueue  Capacity=inf  StatNumberInBlock=on
      settings: OutputPortMap=o1
  IN_Resource : PathCombiner  NumberInputPorts=1
  IN_Shipment : PathCombiner  NumberInputPorts=2  StatLastArrivalPort=on
      settings: OutputPortMap=o1
  Infinite Server : InfiniteServer  ServiceTimeFrom=Signal port t
  Infinite Server1 : InfiniteServer  ServiceTimeFrom=Signal port t
  Mux : Mux  Inputs=3
  N-Server : NServer  NumberOfServers=inf  ServiceTimeFrom=Signal port t  StatNumberInBlock=on
      settings: OutputPortMap=o1
  N-Server1 : NServer  NumberOfServers=inf  ServiceTimeFrom=Signal port t  StatNumberDeparted=on  StatNumberInBlock=on
      settings: OutputPortMap=o0,o1
  OUT_Resource : OutputSwitch  NumberOutputPorts=1
  OUT_Shipment : OutputSwitch  NumberOutputPorts=2  SwitchingCriterion=From signal port p
  Output Switch : OutputSwitch  NumberOutputPorts=2  SwitchingCriterion=From signal port p
  Path Combiner : PathCombiner  NumberInputPorts=2  StatLastArrivalPort=on
      settings: OutputPortMap=o1
  Single Server : SingleServer  ServiceTime=0  StatNumberInBlock=on
      settings: OutputPortMap=o1
  Single Server1 : SingleServer  ServiceTime=0  StatNumberInBlock=on
      settings: OutputPortMap=o1
  Single Server2 : SingleServer  ServiceTime=0
  Single Server3 : SingleServer  ServiceTime=0
  Sum : Sum  Inputs=|++
  Sum1 : Sum  Inputs=|++
  Timed to Event Signal : TimedToEventSignal
  OUT_Shipment_2 : PMIOPort  Port=1  Side=Right
  IN_Shipment_2 : PMIOPort  Port=2  Side=Left
  OUT_Shipment_1 : PMIOPort  Port=3  Side=Left
  IN_Shipment_1 : PMIOPort  Port=4  Side=Right
  In_Resource_1 : PMIOPort  Port=5  Side=Right
  Out_Resource_1 : PMIOPort  Port=6  Side=Right
  tag scope: TC1_Metrics=global
  wires:
  FIFO Queue1/1 -> Sum/2
  FIFO Queue/1 -> Sum/1
  Sum/1 -> Mux/1
  Constant/1 -> Timed to Event Signal/1
  Timed to Event Signal/1 -> Infinite Server/1, N-Server/1, Infinite Server1/1, N-Server1/1
  N-Server/1 -> Sum1/1
  N-Server1/2 -> Sum1/2
  Sum1/1 -> Mux/2
  Mux/1 -> [TC1_Metrics], Discrete Event Signal to Workspace/1
  N-Server1/1 -> Mux/3
  IN_Shipment/1 -> Output Switch/1
  Single Server/1 -> Enabled Gate/1
  Single Server1/1 -> Enabled Gate1/1
  Path Combiner/1 -> OUT_Shipment/1
  connections:
  FIFO Queue/RConn1 -- Enabled Gate/LConn1
  Enabled Gate1/LConn1 -- FIFO Queue1/RConn1
  Infinite Server/LConn1 -- Enabled Gate1/RConn1
  Enabled Gate/RConn1 -- Infinite Server1/LConn1
  Single Server/RConn1 -- N-Server/LConn1
  N-Server/RConn1 -- Single Server1/LConn1
  Single Server1/RConn1 -- N-Server1/LConn1
  IN_Shipment/RConn1 -- Single Server2/LConn1
  Single Server2/RConn1 -- Output Switch/LConn1
  Output Switch/RConn1 -- FIFO Queue/LConn1
  Output Switch/RConn2 -- FIFO Queue1/LConn1
  In_Resource_1/RConn1 -- IN_Resource/LConn1
  IN_Resource/RConn1 -- Single Server/LConn1
  N-Server1/RConn1 -- OUT_Resource/LConn1
  OUT_Resource/RConn1 -- Out_Resource_1/RConn1
  IN_Shipment_1/RConn1 -- IN_Shipment/LConn1
  IN_Shipment_2/RConn1 -- IN_Shipment/LConn2
  Path Combiner/RConn1 -- Single Server3/LConn1
  Single Server3/RConn1 -- OUT_Shipment/LConn1
  Infinite Server1/RConn1 -- Path Combiner/LConn1
  Infinite Server/RConn1 -- Path Combiner/LConn2
  OUT_Shipment/RConn1 -- OUT_Shipment_1/RConn1
  OUT_Shipment/RConn2 -- OUT_Shipment_2/RConn1

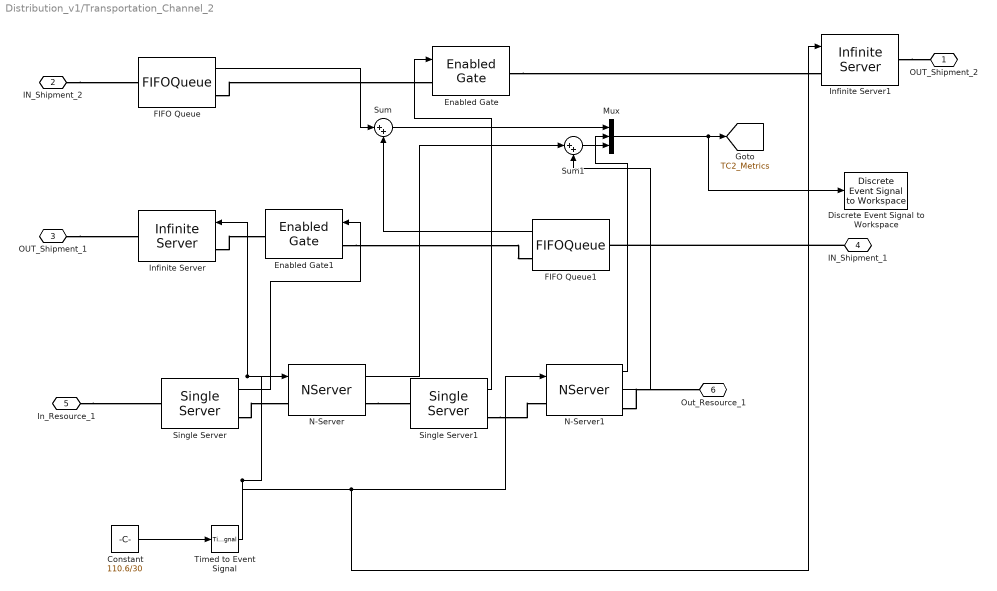
== system Distribution_v1/Transportation_Channel_2 ==
  Constant : Constant  Value=110.6/30
  Discrete Event Signal to Workspace : simeventslib/SimEvents Sinks/Discrete Event Signal to Workspace  VariableName=TC2_Status  SaveFormat=Structure With Time  isMonitorOnly=off  isRecordIC=off
  Enabled Gate : EnabledGate
  Enabled Gate1 : EnabledGate
  FIFO Queue : FIFOQueue  Capacity=inf  StatNumberInBlock=on
      settings: OutputPortMap=o1
  FIFO Queue1 : FIFOQueue  Capacity=inf  StatNumberInBlock=on
      settings: OutputPortMap=o1
  Infinite Server : InfiniteServer  ServiceTimeFrom=Signal port t
  Infinite Server1 : InfiniteServer  ServiceTimeFrom=Signal port t
  Mux : Mux  Inputs=3
  N-Server : NServer  NumberOfServers=inf  ServiceTimeFrom=Signal port t  StatNumberInBlock=on
      settings: OutputPortMap=o1
  N-Server1 : NServer  NumberOfServers=inf  ServiceTimeFrom=Signal port t  StatNumberDeparted=on  StatNumberInBlock=on
      settings: OutputPortMap=o0,o1
  Single Server : SingleServer  ServiceTime=0  StatNumberInBlock=on
      settings: OutputPortMap=o1
  Single Server1 : SingleServer  ServiceTime=0  StatNumberInBlock=on
      settings: OutputPortMap=o1
  Sum : Sum  Inputs=|++
  Sum1 : Sum  Inputs=|++
  Timed to Event Signal : TimedToEventSignal
  OUT_Shipment_2 : PMIOPort  Port=1  Side=Right
  IN_Shipment_2 : PMIOPort  Port=2  Side=Left
  OUT_Shipment_1 : PMIOPort  Port=3  Side=Left
  IN_Shipment_1 : PMIOPort  Port=4  Side=Right
  In_Resource_1 : PMIOPort  Port=5  Side=Right
  Out_Resource_1 : PMIOPort  Port=6  Side=Right
  tag scope: TC2_Metrics=global
  wires:
  FIFO Queue1/1 -> Sum/2
  FIFO Queue/1 -> Sum/1
  Sum/1 -> Mux/1
  Constant/1 -> Timed to Event Signal/1
  Timed to Event Signal/1 -> Infinite Server/1, N-Server/1, Infinite Server1/1, N-Server1/1
  Single Server/1 -> Enabled Gate1/1
  Single Server1/1 -> Enabled Gate/1
  N-Server/1 -> Sum1/1
  Sum1/1 -> Mux/2
  Mux/1 -> [TC2_Metrics], Discrete Event Signal to Workspace/1
  N-Server1/2 -> Sum1/2
  N-Server1/1 -> Mux/3
  connections:
  FIFO Queue/RConn1 -- Enabled Gate/LConn1
  Enabled Gate1/LConn1 -- FIFO Queue1/RConn1
  IN_Shipment_2/RConn1 -- FIFO Queue/LConn1
  IN_Shipment_1/RConn1 -- FIFO Queue1/LConn1
  OUT_Shipment_1/RConn1 -- Infinite Server/RConn1
  Infinite Server/LConn1 -- Enabled Gate1/RConn1
  Infinite Server1/RConn1 -- OUT_Shipment_2/RConn1
  N-Server1/RConn1 -- Out_Resource_1/RConn1
  Enabled Gate/RConn1 -- Infinite Server1/LConn1
  In_Resource_1/RConn1 -- Single Server/LConn1
  Single Server/RConn1 -- N-Server/LConn1
  N-Server/RConn1 -- Single Server1/LConn1
  Single Server1/RConn1 -- N-Server1/LConn1

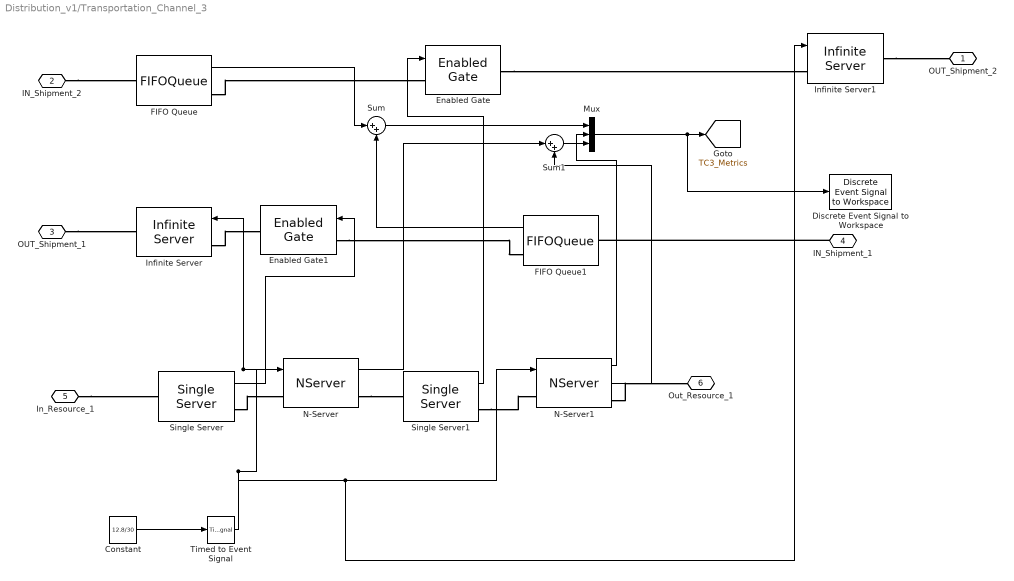
== system Distribution_v1/Transportation_Channel_3 ==
  Constant : Constant  Value=12.8/30
  Discrete Event Signal to Workspace : simeventslib/SimEvents Sinks/Discrete Event Signal to Workspace  VariableName=TC3_Status  SaveFormat=Structure With Time  isMonitorOnly=off  isRecordIC=off
  Enabled Gate : EnabledGate
  Enabled Gate1 : EnabledGate
  FIFO Queue : FIFOQueue  Capacity=inf  StatNumberInBlock=on
      settings: OutputPortMap=o1
  FIFO Queue1 : FIFOQueue  Capacity=inf  StatNumberInBlock=on
      settings: OutputPortMap=o1
  Infinite Server : InfiniteServer  ServiceTimeFrom=Signal port t
  Infinite Server1 : InfiniteServer  ServiceTimeFrom=Signal port t
  Mux : Mux  Inputs=3
  N-Server : NServer  NumberOfServers=inf  ServiceTimeFrom=Signal port t  StatNumberInBlock=on
      settings: OutputPortMap=o1
  N-Server1 : NServer  NumberOfServers=inf  ServiceTimeFrom=Signal port t  StatNumberDeparted=on  StatNumberInBlock=on
      settings: OutputPortMap=o0,o1
  Single Server : SingleServer  ServiceTime=0  StatNumberInBlock=on
      settings: OutputPortMap=o1
  Single Server1 : SingleServer  ServiceTime=0  StatNumberInBlock=on
      settings: OutputPortMap=o1
  Sum : Sum  Inputs=|++
  Sum1 : Sum  Inputs=|++
  Timed to Event Signal : TimedToEventSignal
  OUT_Shipment_2 : PMIOPort  Port=1  Side=Right
  IN_Shipment_2 : PMIOPort  Port=2  Side=Left
  OUT_Shipment_1 : PMIOPort  Port=3  Side=Left
  IN_Shipment_1 : PMIOPort  Port=4  Side=Right
  In_Resource_1 : PMIOPort  Port=5  Side=Right
  Out_Resource_1 : PMIOPort  Port=6  Side=Right
  tag scope: TC3_Metrics=global
  wires:
  FIFO Queue1/1 -> Sum/2
  FIFO Queue/1 -> Sum/1
  Constant/1 -> Timed to Event Signal/1
  Timed to Event Signal/1 -> Infinite Server/1, N-Server/1, Infinite Server1/1, N-Server1/1
  Single Server/1 -> Enabled Gate1/1
  Single Server1/1 -> Enabled Gate/1
  N-Server/1 -> Sum1/1
  N-Server1/2 -> Sum1/2
  Sum1/1 -> Mux/2
  Mux/1 -> [TC3_Metrics], Discrete Event Signal to Workspace/1
  Sum/1 -> Mux/1
  N-Server1/1 -> Mux/3
  connections:
  FIFO Queue/RConn1 -- Enabled Gate/LConn1
  Enabled Gate1/LConn1 -- FIFO Queue1/RConn1
  IN_Shipment_2/RConn1 -- FIFO Queue/LConn1
  IN_Shipment_1/RConn1 -- FIFO Queue1/LConn1
  OUT_Shipment_1/RConn1 -- Infinite Server/RConn1
  Infinite Server/LConn1 -- Enabled Gate1/RConn1
  Infinite Server1/RConn1 -- OUT_Shipment_2/RConn1
  N-Server1/RConn1 -- Out_Resource_1/RConn1
  Enabled Gate/RConn1 -- Infinite Server1/LConn1
  In_Resource_1/RConn1 -- Single Server/LConn1
  Single Server/RConn1 -- N-Server/LConn1
  N-Server/RConn1 -- Single Server1/LConn1
  Single Server1/RConn1 -- N-Server1/LConn1

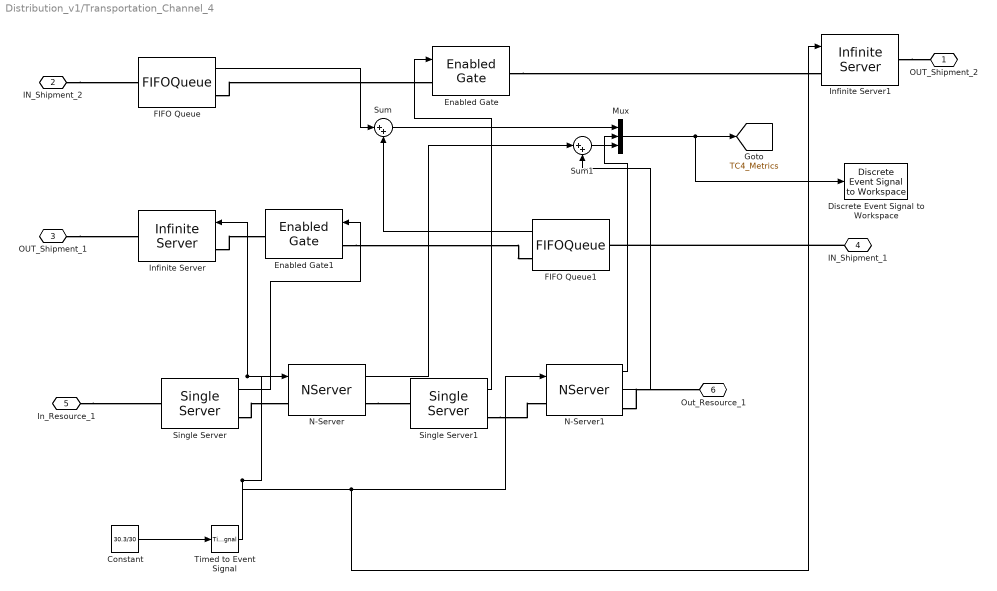
== system Distribution_v1/Transportation_Channel_4 ==
  Constant : Constant  Value=30.3/30
  Discrete Event Signal to Workspace : simeventslib/SimEvents Sinks/Discrete Event Signal to Workspace  VariableName=TC4_Status  SaveFormat=Structure With Time  isMonitorOnly=off  isRecordIC=off
  Enabled Gate : EnabledGate
  Enabled Gate1 : EnabledGate
  FIFO Queue : FIFOQueue  Capacity=inf  StatNumberInBlock=on
      settings: OutputPortMap=o1
  FIFO Queue1 : FIFOQueue  Capacity=inf  StatNumberInBlock=on
      settings: OutputPortMap=o1
  Infinite Server : InfiniteServer  ServiceTimeFrom=Signal port t
  Infinite Server1 : InfiniteServer  ServiceTimeFrom=Signal port t
  Mux : Mux  Inputs=3
  N-Server : NServer  NumberOfServers=inf  ServiceTimeFrom=Signal port t  StatNumberInBlock=on
      settings: OutputPortMap=o1
  N-Server1 : NServer  NumberOfServers=inf  ServiceTimeFrom=Signal port t  StatNumberDeparted=on  StatNumberInBlock=on
      settings: OutputPortMap=o0,o1
  Single Server : SingleServer  ServiceTime=0  StatNumberInBlock=on
      settings: OutputPortMap=o1
  Single Server1 : SingleServer  ServiceTime=0  StatNumberInBlock=on
      settings: OutputPortMap=o1
  Sum : Sum  Inputs=|++
  Sum1 : Sum  Inputs=|++
  Timed to Event Signal : TimedToEventSignal
  OUT_Shipment_2 : PMIOPort  Port=1  Side=Right
  IN_Shipment_2 : PMIOPort  Port=2  Side=Left
  OUT_Shipment_1 : PMIOPort  Port=3  Side=Left
  IN_Shipment_1 : PMIOPort  Port=4  Side=Right
  In_Resource_1 : PMIOPort  Port=5  Side=Right
  Out_Resource_1 : PMIOPort  Port=6  Side=Right
  tag scope: TC4_Metrics=global
  wires:
  FIFO Queue1/1 -> Sum/2
  FIFO Queue/1 -> Sum/1
  Constant/1 -> Timed to Event Signal/1
  Timed to Event Signal/1 -> Infinite Server/1, N-Server/1, Infinite Server1/1, N-Server1/1
  Single Server/1 -> Enabled Gate1/1
  Single Server1/1 -> Enabled Gate/1
  Sum/1 -> Mux/1
  N-Server/1 -> Sum1/1
  N-Server1/2 -> Sum1/2
  Sum1/1 -> Mux/2
  Mux/1 -> [TC4_Metrics], Discrete Event Signal to Workspace/1
  N-Server1/1 -> Mux/3
  connections:
  FIFO Queue/RConn1 -- Enabled Gate/LConn1
  Enabled Gate1/LConn1 -- FIFO Queue1/RConn1
  IN_Shipment_2/RConn1 -- FIFO Queue/LConn1
  IN_Shipment_1/RConn1 -- FIFO Queue1/LConn1
  OUT_Shipment_1/RConn1 -- Infinite Server/RConn1
  Infinite Server/LConn1 -- Enabled Gate1/RConn1
  Infinite Server1/RConn1 -- OUT_Shipment_2/RConn1
  N-Server1/RConn1 -- Out_Resource_1/RConn1
  Enabled Gate/RConn1 -- Infinite Server1/LConn1
  In_Resource_1/RConn1 -- Single Server/LConn1
  Single Server/RConn1 -- N-Server/LConn1
  N-Server/RConn1 -- Single Server1/LConn1
  Single Server1/RConn1 -- N-Server1/LConn1

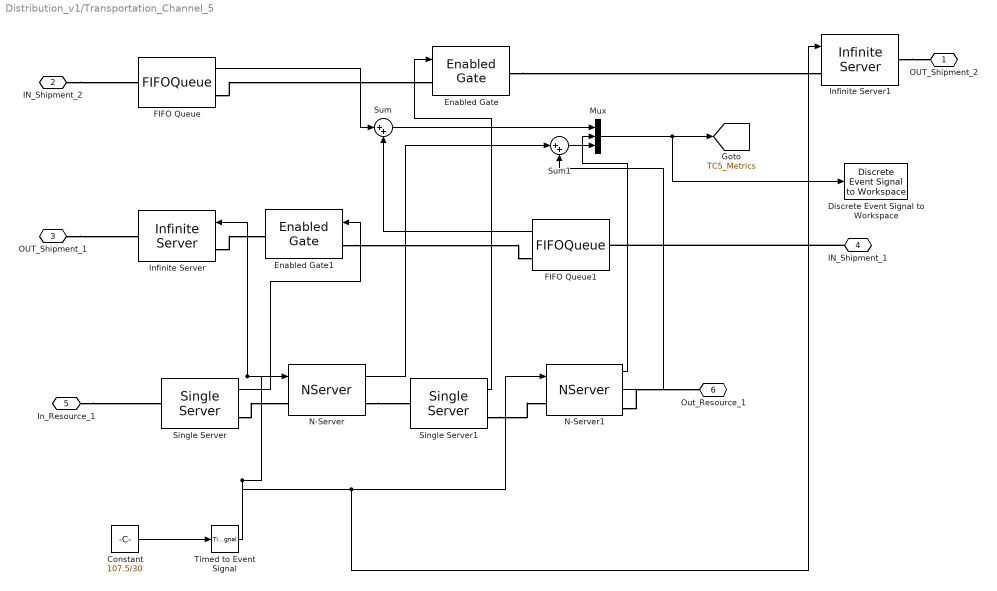
== system Distribution_v1/Transportation_Channel_5 ==
  Constant : Constant  Value=107.5/30
  Discrete Event Signal to Workspace : simeventslib/SimEvents Sinks/Discrete Event Signal to Workspace  VariableName=TC5_Status  SaveFormat=Structure With Time  isMonitorOnly=off  isRecordIC=off
  Enabled Gate : EnabledGate
  Enabled Gate1 : EnabledGate
  FIFO Queue : FIFOQueue  Capacity=inf  StatNumberInBlock=on
      settings: OutputPortMap=o1
  FIFO Queue1 : FIFOQueue  Capacity=inf  StatNumberInBlock=on
      settings: OutputPortMap=o1
  Infinite Server : InfiniteServer  ServiceTimeFrom=Signal port t
  Infinite Server1 : InfiniteServer  ServiceTimeFrom=Signal port t
  Mux : Mux  Inputs=3
  N-Server : NServer  NumberOfServers=inf  ServiceTimeFrom=Signal port t  StatNumberInBlock=on
      settings: OutputPortMap=o1
  N-Server1 : NServer  NumberOfServers=inf  ServiceTimeFrom=Signal port t  StatNumberDeparted=on  StatNumberInBlock=on
      settings: OutputPortMap=o0,o1
  Single Server : SingleServer  ServiceTime=0  StatNumberInBlock=on
      settings: OutputPortMap=o1
  Single Server1 : SingleServer  ServiceTime=0  StatNumberInBlock=on
      settings: OutputPortMap=o1
  Sum : Sum  Inputs=|++
  Sum1 : Sum  Inputs=|++
  Timed to Event Signal : TimedToEventSignal
  OUT_Shipment_2 : PMIOPort  Port=1  Side=Right
  IN_Shipment_2 : PMIOPort  Port=2  Side=Left
  OUT_Shipment_1 : PMIOPort  Port=3  Side=Left
  IN_Shipment_1 : PMIOPort  Port=4  Side=Right
  In_Resource_1 : PMIOPort  Port=5  Side=Right
  Out_Resource_1 : PMIOPort  Port=6  Side=Right
  tag scope: TC5_Metrics=global
  wires:
  FIFO Queue1/1 -> Sum/2
  FIFO Queue/1 -> Sum/1
  Constant/1 -> Timed to Event Signal/1
  Timed to Event Signal/1 -> Infinite Server/1, N-Server/1, Infinite Server1/1, N-Server1/1
  Single Server/1 -> Enabled Gate1/1
  Single Server1/1 -> Enabled Gate/1
  Sum/1 -> Mux/1
  N-Server/1 -> Sum1/1
  N-Server1/2 -> Sum1/2
  Sum1/1 -> Mux/2
  Mux/1 -> [TC5_Metrics], Discrete Event Signal to Workspace/1
  N-Server1/1 -> Mux/3
  connections:
  FIFO Queue/RConn1 -- Enabled Gate/LConn1
  Enabled Gate1/LConn1 -- FIFO Queue1/RConn1
  IN_Shipment_2/RConn1 -- FIFO Queue/LConn1
  IN_Shipment_1/RConn1 -- FIFO Queue1/LConn1
  OUT_Shipment_1/RConn1 -- Infinite Server/RConn1
  Infinite Server/LConn1 -- Enabled Gate1/RConn1
  Infinite Server1/RConn1 -- OUT_Shipment_2/RConn1
  N-Server1/RConn1 -- Out_Resource_1/RConn1
  Enabled Gate/RConn1 -- Infinite Server1/LConn1
  In_Resource_1/RConn1 -- Single Server/LConn1
  Single Server/RConn1 -- N-Server/LConn1
  N-Server/RConn1 -- Single Server1/LConn1
  Single Server1/RConn1 -- N-Server1/LConn1

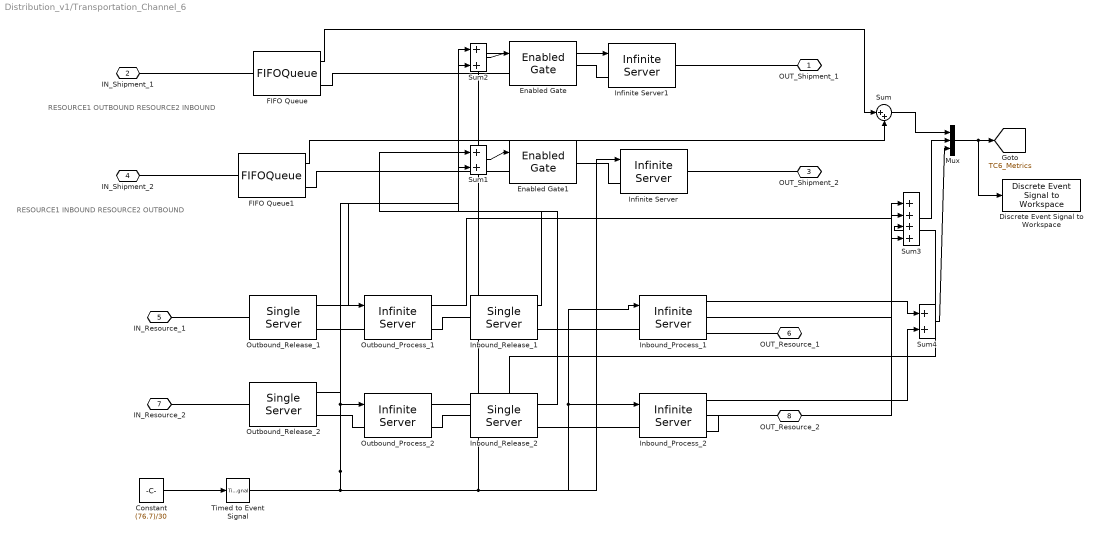
== system Distribution_v1/Transportation_Channel_6 ==
  note: RESOURCE1 INBOUND
      | RESOURCE2 OUTBOUND
  note: RESOURCE1 OUTBOUND
      | RESOURCE2 INBOUND
  Constant : Constant  Value=(76.7)/30
  Discrete Event Signal to Workspace : simeventslib/SimEvents Sinks/Discrete Event Signal to Workspace  VariableName=TC6_Status  SaveFormat=Structure With Time  isMonitorOnly=off  isRecordIC=off
  Enabled Gate : EnabledGate
  Enabled Gate1 : EnabledGate
  FIFO Queue : FIFOQueue  Capacity=inf  StatNumberInBlock=on
      settings: OutputPortMap=o1
  FIFO Queue1 : FIFOQueue  Capacity=inf  StatNumberInBlock=on
      settings: OutputPortMap=o1
  Inbound_Process_1 : InfiniteServer  ServiceTimeFrom=Signal port t  ServiceTime=(76.7)/30  StatNumberDeparted=on  StatNumberInBlock=on
      settings: OutputPortMap=o0,o1
  Inbound_Process_2 : InfiniteServer  ServiceTimeFrom=Signal port t  ServiceTime=(76.7)/30  StatNumberDeparted=on  StatNumberInBlock=on
      settings: OutputPortMap=o0,o1
  Inbound_Release_1 : SingleServer  ServiceTime=0  StatNumberInBlock=on
      settings: OutputPortMap=o1
  Inbound_Release_2 : SingleServer  ServiceTime=0  StatNumberInBlock=on
      settings: OutputPortMap=o1
  Infinite Server : InfiniteServer  ServiceTimeFrom=Signal port t  ServiceTime=(76.7)/30
  Infinite Server1 : InfiniteServer  ServiceTimeFrom=Signal port t  ServiceTime=(76.7)/30
  Mux : Mux  Inputs=3
  Outbound_Process_1 : InfiniteServer  ServiceTimeFrom=Signal port t  ServiceTime=(76.7)/30  StatNumberInBlock=on
      settings: OutputPortMap=o1
  Outbound_Process_2 : InfiniteServer  ServiceTimeFrom=Signal port t  ServiceTime=(76.7)/30  StatNumberInBlock=on
      settings: OutputPortMap=o1
  Outbound_Release_1 : SingleServer  ServiceTime=0  StatNumberInBlock=on
      settings: OutputPortMap=o1
  Outbound_Release_2 : SingleServer  ServiceTime=0  StatNumberInBlock=on
      settings: OutputPortMap=o1
  Sum{,1..2,4} (4 alike) : Sum  Inputs=|++
  Sum3 : Sum  Inputs=|++++
  Timed to Event Signal : TimedToEventSignal
  OUT_Shipment_1 : PMIOPort  Port=1  Side=Right
  IN_Shipment_1 : PMIOPort  Port=2  Side=Right
  OUT_Shipment_2 : PMIOPort  Port=3  Side=Left
  IN_Shipment_2 : PMIOPort  Port=4  Side=Left
  IN_Resource_1 : PMIOPort  Port=5  Side=Right
  OUT_Resource_1 : PMIOPort  Port=6  Side=Right
  IN_Resource_2 : PMIOPort  Port=7  Side=Left
  OUT_Resource_2 : PMIOPort  Port=8  Side=Left
  tag scope: TC6_Metrics=global
  wires:
  FIFO Queue1/1 -> Sum/2
  FIFO Queue/1 -> Sum/1
  Constant/1 -> Timed to Event Signal/1
  Timed to Event Signal/1 -> Outbound_Process_1/1, Outbound_Process_2/1, Infinite Server1/1, Inbound_Process_1/1, Inbound_Process_2/1, Infinite Server/1
  Sum1/1 -> Enabled Gate1/1
  Outbound_Release_2/1 -> Sum1/2
  Inbound_Release_1/1 -> Sum1/1
  Sum2/1 -> Enabled Gate/1
  Outbound_Release_1/1 -> Sum2/1
  Inbound_Release_2/1 -> Sum2/2
  Mux/1 -> [TC6_Metrics], Discrete Event Signal to Workspace/1
  Sum/1 -> Mux/1
  Sum3/1 -> Mux/2
  Outbound_Process_1/1 -> Sum3/1
  Inbound_Process_1/2 -> Sum3/2
  Outbound_Process_2/1 -> Sum3/3
  Inbound_Process_2/2 -> Sum3/4
  Inbound_Process_1/1 -> Sum4/1
  Inbound_Process_2/1 -> Sum4/2
  Sum4/1 -> Mux/3
  connections:
  FIFO Queue/RConn1 -- Enabled Gate/LConn1
  Enabled Gate1/LConn1 -- FIFO Queue1/RConn1
  IN_Shipment_1/RConn1 -- FIFO Queue/LConn1
  IN_Shipment_2/RConn1 -- FIFO Queue1/LConn1
  IN_Resource_1/RConn1 -- Outbound_Release_1/LConn1
  OUT_Shipment_2/RConn1 -- Infinite Server/RConn1
  Infinite Server/LConn1 -- Enabled Gate1/RConn1
  Enabled Gate/RConn1 -- Infinite Server1/LConn1
  Infinite Server1/RConn1 -- OUT_Shipment_1/RConn1
  IN_Resource_2/RConn1 -- Outbound_Release_2/LConn1
  Outbound_Release_2/RConn1 -- Outbound_Process_2/LConn1
  Outbound_Process_2/RConn1 -- Inbound_Release_2/LConn1
  Inbound_Release_2/RConn1 -- Inbound_Process_2/LConn1
  Inbound_Process_2/RConn1 -- OUT_Resource_2/RConn1
  Outbound_Release_1/RConn1 -- Outbound_Process_1/LConn1
  Inbound_Release_1/RConn1 -- Inbound_Process_1/LConn1
  Outbound_Process_1/RConn1 -- Inbound_Release_1/LConn1
  Inbound_Process_1/RConn1 -- OUT_Resource_1/RConn1
